simulink model "park_transform_cosim_verification"  (Simulink 6.4)
settings: Solver=FixedStepDiscrete  StartTime=0.0  StopTime=1e-1  FixedStep=1e-4  RelTol=1e-3
undefined symbols (not defined in the file or in its folder): pipeline_prec
libraries: modelsimlib x1, powerlib_extras x1, simulink x1
settings Model: LastModifiedBy=Administrador

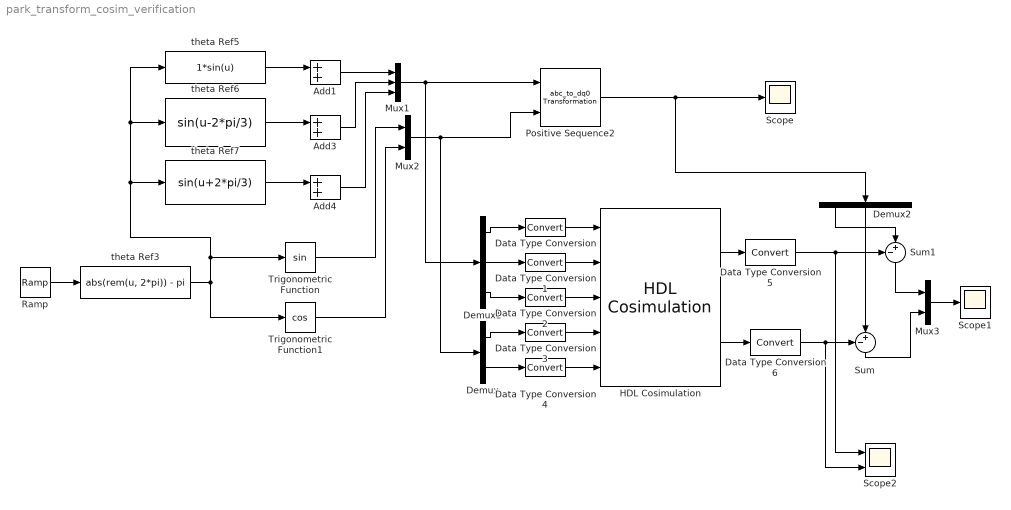
== system park_transform_cosim_verification ==
  Add1 : Sum  OutScaling=2^-10
  Add3 : Sum  OutScaling=2^-10
  Add4 : Sum  OutScaling=2^-10
  Data Type Conversion{,1..4} (5 alike) : DataTypeConversion  OutDataTypeMode=Specify via dialog  OutScaling=2^(-pipeline_prec)  RndMeth=Nearest  SaturateOnIntegerOverflow=on
  Data Type Conversion5 : DataTypeConversion
  Data Type Conversion6 : DataTypeConversion
  Demux : Demux  Outputs=2
  Demux1 : Demux  Outputs=3
  Demux2 : Demux  Orientation=down  Outputs=3
  HDL Cosimulation : modelsimlib/HDL Cosimulation  DialogController=modelsimddg.CoSim  DialogControllerArgs=DataTag0  PortPaths=park_transform_wrapper/a;park_transform_wrapper/b;park_transform_wrapper/c;park_transform_wrapper/sin;park_transform_wrapper/cos;park_transform_wrapper/d;park_transform_wrapper/q  PortModes=[1 1 1 1 1 2 2 ]  PortTimes=[1,1,1,1,1,1e-4,1e-4]  PortSigns=[-1 -1 -1 -1 -1 1 1 ]  PortFracLengths=[0,0,0,0,0,pipeline_prec,pipeline_prec]  CommLocal=on  CommSharedMemory=off  CommPortNumber=4449  CommShowInfo=off  ClockModes=[]  ClockTimes=[]  TclPreSimCommand="echo \"Running Simulink Cosimulation block.\""  TclPostSimCommand="echo \"done\""  TimingMode=s  TimingScaleFactor=1  idxCellArray={'UNUSED_VAR'}
  Mux1 : Mux  Inputs=3
  Mux2 : Mux  Inputs=2
  Mux3 : Mux  Inputs=2
  Positive Sequence2 : powerlib_extras/Measurements/abc_to_dq0 Transformation  SystemSampleTime=-1
  Ramp : simulink/Sources/Ramp  SystemSampleTime=-1  slope=2*pi*50  start=0  X0=0
  Scope : Scope
  Scope1 : Scope
  Scope2 : Scope  NumInputPorts=2
      settings: YMin=0.99925~-5  YMax=1.00025~5  SaveName=ScopeData2
  Sum : Sum  Orientation=down  Inputs=-+|
  Sum1 : Sum  Orientation=down  Inputs=-+|
  Trigonometric Function : Trigonometry
  Trigonometric Function1 : Trigonometry  Operator=cos
  theta Ref3 : Fcn  Expr=abs(rem(u, 2*pi)) - pi  SampleTime=1e-4
  theta Ref5 : Fcn  Expr=1*sin(u)
  theta Ref6 : Fcn  Expr=sin(u-2*pi/3)
  theta Ref7 : Fcn  Expr=sin(u+2*pi/3)
  wires:
  Ramp/1 -> theta Ref3/1
  theta Ref3/1 -> theta Ref5/1, theta Ref6/1, theta Ref7/1, Trigonometric Function/1, Trigonometric Function1/1
  theta Ref5/1 -> Add1/1
  theta Ref6/1 -> Add3/1
  theta Ref7/1 -> Add4/1
  Add4/1 -> Mux1/3
  Add3/1 -> Mux1/2
  Add1/1 -> Mux1/1
  Mux1/1 -> Positive Sequence2/1, Demux1/1
  Mux2/1 -> Positive Sequence2/2, Demux/1
  Trigonometric Function/1 -> Mux2/1
  Trigonometric Function1/1 -> Mux2/2
  Positive Sequence2/1 -> Scope/1, Demux2/1
  Demux1/1 -> Data Type Conversion/1
  Data Type Conversion/1 -> HDL Cosimulation/1
  Data Type Conversion2/1 -> HDL Cosimulation/3
  Data Type Conversion1/1 -> HDL Cosimulation/2
  Demux1/2 -> Data Type Conversion1/1
  Demux1/3 -> Data Type Conversion2/1
  Demux/1 -> Data Type Conversion3/1
  Data Type Conversion3/1 -> HDL Cosimulation/4
  Data Type Conversion4/1 -> HDL Cosimulation/5
  Demux/2 -> Data Type Conversion4/1
  HDL Cosimulation/1 -> Data Type Conversion5/1
  HDL Cosimulation/2 -> Data Type Conversion6/1
  Data Type Conversion5/1 -> Sum1/1, Scope2/1
  Data Type Conversion6/1 -> Sum/1, Scope2/2
  Demux2/1 -> Sum1/2
  Sum1/1 -> Mux3/1
  Sum/1 -> Mux3/2
  Mux3/1 -> Scope1/1
  Demux2/2 -> Sum/2
